simulink model "EEG_2022_040_Simulink_ex3"  (R2024a)
settings: Solver=VariableStepAuto  StartTime=0.0  StopTime=50  RelTol=1e-3
settings Model: Creator=User  LastModifiedBy=User

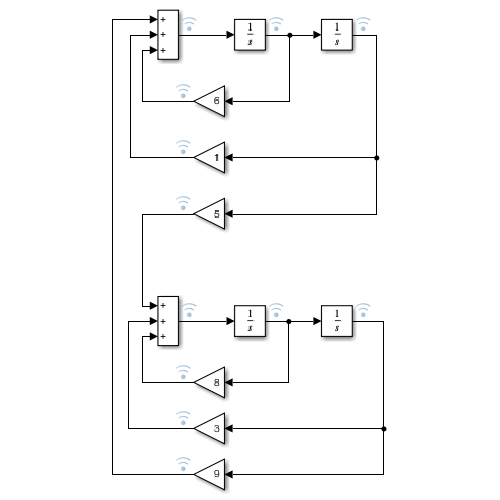
[thumbnail: Simulink's stored preview of the top-level diagram]
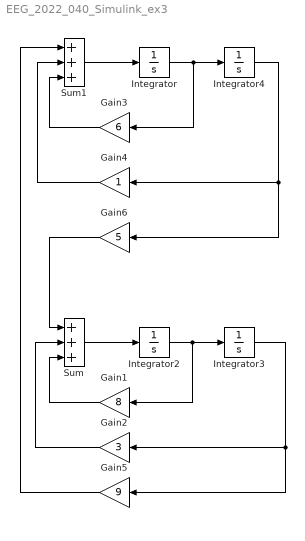
== system EEG_2022_040_Simulink_ex3 ==
  Gain1 : Gain  Gain=8
  Gain2 : Gain  Gain=3
  Gain3 : Gain  Gain=6
  Gain4 : Gain
  Gain5 : Gain  Gain=9
  Gain6 : Gain  Gain=5
  Integrator{,2..4} (4 alike) : Integrator
  Sum : Sum  Inputs=+++
  Sum1 : Sum  Inputs=+++
  wires:
  Sum1/1 -> Integrator/1
  Integrator/1 -> Integrator4/1, Gain3/1
  Gain3/1 -> Sum1/3
  Integrator4/1 -> Gain6/1, Gain4/1
  Integrator3/1 -> Gain5/1, Gain2/1
  Gain6/1 -> Sum/1
  Gain4/1 -> Sum1/2
  Integrator2/1 -> Integrator3/1, Gain1/1
  Sum/1 -> Integrator2/1
  Gain5/1 -> Sum1/1
  Gain1/1 -> Sum/3
  Gain2/1 -> Sum/2
